simulink model "current_feedback"  (R2023b)
settings: Solver=VariableStepAuto  StartTime=0.0  StopTime=10.0  RelTol=1e-3
libraries: cstblocks x2
settings Model: Creator=frenci  LastModifiedBy=frenci

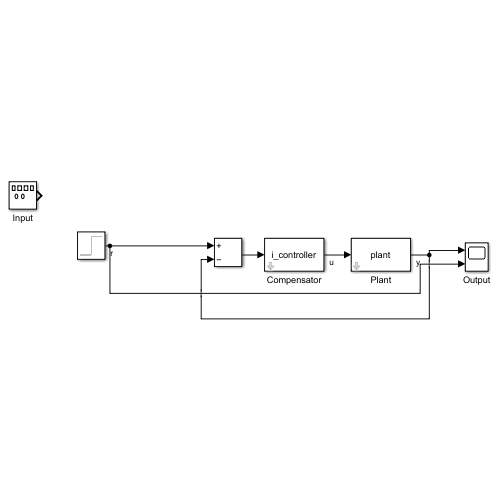
[thumbnail: Simulink's stored preview of the top-level diagram]
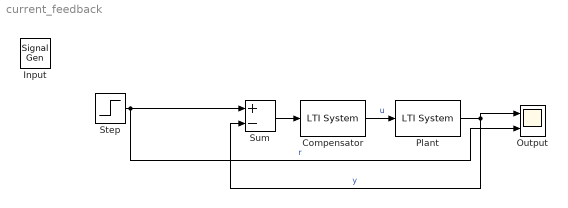
== system current_feedback ==
  Compensator : cstblocks/LTI System  sys=i_controller  IC=[]  PadeOrder=0
  Input : SignalGenerator
  Output : Scope  NumInputPorts=2
  Plant : cstblocks/LTI System  sys=plant  IC=[]  PadeOrder=0
  Step : Step  SampleTime=0
  Sum : Sum  Inputs=+-
  wires:
  Step/1 -> Sum/1, Output/2  "r"
  Sum/1 -> Compensator/1
  Compensator/1 -> Plant/1  "u"
  Plant/1 -> Sum/2, Output/1  "y"
